simulink model "radarDFT"  (R2013a)
settings: Solver=ode45  StartTime=0.0  StopTime=90  RelTol=1e-3
PostLoadFcn:
  | bps_model_init(gcs);
undefined symbols (not defined in the file): xlipgetpartsetting
libraries: xbsIndex_r4 x69, xps_library x25, mbee4_library x4
(part 3 of 3)

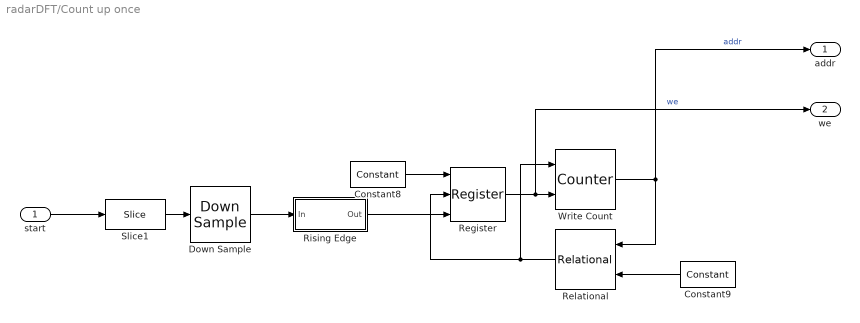
== system radarDFT/Count up once ==
  start : Inport
  Constant8 : xbsIndex_r4/Constant  const=1  gui_display_data_type=Fixed-point  arith_type=Boolean  n_bits=1  bin_pt=0  preci_type=Single  exp_width=8  frac_width=24  explicit_period=off  period=1  equ=P=C  opselect=C  inp2=PCIN>>17  opr=+  inp1=P  carry=CIN  dbl_ovrd=off  block_type=constant
  Constant9 : xbsIndex_r4/Constant  const=str2num(get_param('radarDFT/numofsamples','value'))-2  gui_display_data_type=Fixed-point  arith_type=Unsigned  n_bits=19  bin_pt=0  preci_type=Single  exp_width=8  frac_width=24  explicit_period=off  period=1e-8  equ=P=C  opselect=C  inp2=PCIN>>17  opr=+  inp1=P  carry=CIN  dbl_ovrd=off  block_type=constant
  Down Sample : xbsIndex_r4/Down Sample  sample_ratio=fix(250000/str2num(get_param('radarDFT/sampfreq(kHz)','value')))  sample_phase="Last Value of Frame  (most efficient)"  en=off  latency=1  dbl_ovrd=off  block_type=dsamp
  Register : xbsIndex_r4/Register  init=0  rst=on  en=on  dbl_ovrd=off  block_type=register
  Relational : xbsIndex_r4/Relational  mode=a=b  en=off  latency=1  dbl_ovrd=off  block_type=relational
      settings: block_version=10.1.3
  Rising Edge : Subsystem
  Slice1 : xbsIndex_r4/Slice  nbits=1  boolean_output=on  mode=Lower Bit Location + Width  bit1=0  base1=MSB of Input  bit0=0  base0=LSB of Input  dbl_ovrd=off  block_type=slice
      settings: infoedit="Extracts a given range of bits from each input sample and presents it at the output.  The output type is ordinarily unsigned with binary point at zero, but can be Boolean when the slice is one bit wide.<P><P>Hardware notes: In hardware this block costs nothing."  block_version=10.1.3
  Write Count : xbsIndex_r4/Counter  cnt_type=Free Running  cnt_to=Inf  operation=Up  start_count=0  cnt_by_val=1  arith_type=Unsigned  n_bits=19  bin_pt=0  load_pin=off  rst=on  en=on  explicit_period=on  period=fix(250000/str2num(get_param('radarDFT/sampfreq(kHz)','value')))  dbl_ovrd=off  use_behavioral_HDL=off  implementation=Fabric  use_rpm=off  block_type=counter
  addr : Outport
  we : Outport  Port=2
  wires:
  Write Count/1 -> addr/1, Relational/1  "addr"
  Relational/1 -> Write Count/1, Register/2
  Constant9/1 -> Relational/2
  Register/1 -> we/1, Write Count/2  "we"
  Rising Edge/1(Out) -> Register/3
  Slice1/1 -> Down Sample/1
  Constant8/1 -> Register/1
  start/1 -> Slice1/1
  Down Sample/1 -> Rising Edge/1(In)

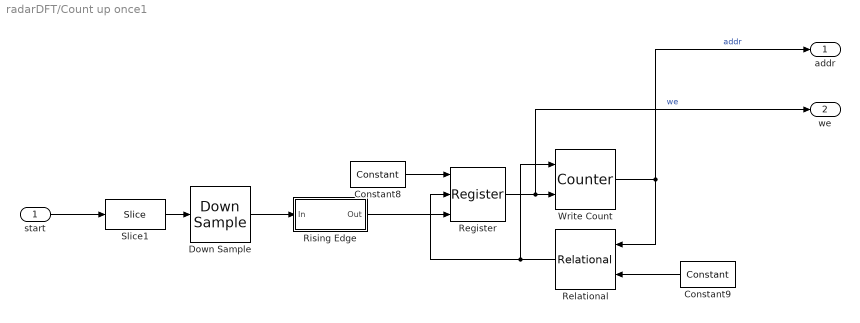
== system radarDFT/Count up once1 ==
  start : Inport
  Constant8 : xbsIndex_r4/Constant  const=1  gui_display_data_type=Boolean  arith_type=Boolean  n_bits=1  bin_pt=0  preci_type=Single  exp_width=8  frac_width=24  explicit_period=off  period=1  equ=P=C  opselect=C  inp2=PCIN>>17  opr=+  inp1=P  carry=CIN  dbl_ovrd=off  block_type=constant
  Constant9 : xbsIndex_r4/Constant  const=2^16-2  gui_display_data_type=Fixed-point  arith_type=Unsigned  n_bits=16  bin_pt=0  preci_type=Single  exp_width=8  frac_width=24  explicit_period=off  period=1e-8  equ=P=C  opselect=C  inp2=PCIN>>17  opr=+  inp1=P  carry=CIN  dbl_ovrd=off  block_type=constant
  Down Sample : xbsIndex_r4/Down Sample  sample_ratio=fix(250000/30)  sample_phase="Last Value of Frame  (most efficient)"  en=off  latency=1  dbl_ovrd=off  block_type=dsamp
  Register : xbsIndex_r4/Register  init=0  rst=on  en=on  dbl_ovrd=off  block_type=register
  Relational : xbsIndex_r4/Relational  mode=a=b  en=off  latency=1  dbl_ovrd=off  block_type=relational
      settings: block_version=10.1.3
  Rising Edge : Subsystem
  Slice1 : xbsIndex_r4/Slice  nbits=1  boolean_output=on  mode=Lower Bit Location + Width  bit1=0  base1=MSB of Input  bit0=0  base0=LSB of Input  dbl_ovrd=off  block_type=slice
      settings: infoedit="Extracts a given range of bits from each input sample and presents it at the output.  The output type is ordinarily unsigned with binary point at zero, but can be Boolean when the slice is one bit wide.<P><P>Hardware notes: In hardware this block costs nothing."  block_version=10.1.3
  Write Count : xbsIndex_r4/Counter  cnt_type=Free Running  cnt_to=Inf  operation=Up  start_count=0  cnt_by_val=1  arith_type=Unsigned  n_bits=16  bin_pt=0  load_pin=off  rst=on  en=on  explicit_period=on  period=fix(250000/30)  dbl_ovrd=off  use_behavioral_HDL=off  implementation=Fabric  use_rpm=off  block_type=counter
  addr : Outport
  we : Outport  Port=2
  wires:
  Write Count/1 -> addr/1, Relational/1  "addr"
  Relational/1 -> Write Count/1, Register/2
  Constant9/1 -> Relational/2
  Register/1 -> we/1, Write Count/2  "we"
  Rising Edge/1(Out) -> Register/3
  Slice1/1 -> Down Sample/1
  Constant8/1 -> Register/1
  start/1 -> Slice1/1
  Down Sample/1 -> Rising Edge/1(In)

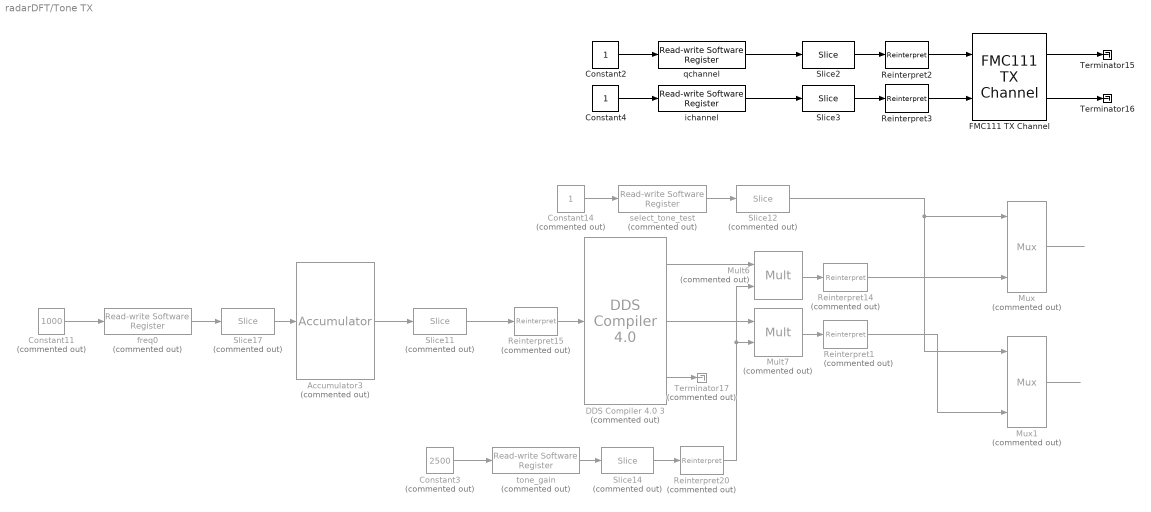
== system radarDFT/Tone TX ==
  Accumulator3 : xbsIndex_r4/Accumulator  Commented=on  operation=Add  n_bits=24  overflow=Wrap  scale=1  rst=off  infoeditControl=reset for floating point data type must be asserted for a minimum of 2 cycles  hasbypass=on  en=off  latency=0  dbl_ovrd=off  msb_inp=100  msb=100  lsb=-100  use_behavioral_HDL=on  implementation=Fabric  block_type=accum
  Constant11 : Constant  Commented=on  Value=1000
  Constant14 : Constant  Commented=on
  Constant2 : Constant
  Constant3 : Constant  Commented=on  Value=2500
  Constant4 : Constant
  DDS Compiler 4.0 3 : xbsIndex_r4/DDS Compiler 4.0   Commented=on  partspresent=SIN_COS_LUT_only  dds_clock_rate=100  channels=1  parameter_entry=Hardware_Parameters  spurious_free_dynamic_range=36  frequency_resolution=0.4  noise_shaping=None  phase_width=16  output_width=16  output_selection=Sine_and_Cosine  negative_sine=off  negative_cosine=off  amplitude_mode=Full_Range  memory_type=Distributed_ROM  optimization_goal=Auto  dsp48_use=Minimal  latency_configuration=Auto  latency=6  has_phase_out=on  sclr_pin=off  clock_enable=off  rfd=off  rdy=off  channel_pin=off  explicit_period=off  period=1  phase_increment=Fixed  output_frequency1=0  output_frequency2=0  output_frequency3=0  output_frequency4=0  output_frequency5=0  output_frequency6=0  output_frequency7=0  output_frequency8=0  output_frequency9=0  output_frequency10=0  output_frequency11=0  output_frequency12=0  output_frequency13=0  output_frequency14=0  output_frequency15=0  output_frequency16=0  pinc1='0'  pinc2='0'  pinc3='0'  pinc4='0'  pinc5='0'  pinc6='0'  pinc7='0'  pinc8='0'  pinc9='0'  pinc10='0'  pinc11='0'  pinc12='0'  pinc13='0'  pinc14='0'  pinc15='0'  pinc16='0'  phase_offset=None  phase_offset_angles1=0  phase_offset_angles2=0  phase_offset_angles3=0  phase_offset_angles4=0  phase_offset_angles5=0  phase_offset_angles6=0  phase_offset_angles7=0  phase_offset_angles8=0  phase_offset_angles9=0  phase_offset_angles10=0  phase_offset_angles11=0  phase_offset_angles12=0  phase_offset_angles13=0  phase_offset_angles14=0  phase_offset_angles15=0  phase_offset_angles16=0  poff1='0'  poff2='0'  poff3='0'  poff4='0'  poff5='0'  poff6='0'  poff7='0'  poff8='0'  poff9='0'  poff10='0'  poff11='0'  poff12='0'  poff13='0'  poff14='0'  poff15='0'  poff16='0'  por_mode=false  gui_behaviour=Sysgen  ip_name=DDS Compiler  ip_version=4.0  dsptool_ready=true  wrapper_available=true  port_translation_map={ 'ce' => 'en', 'sclr' => 'rst' }  ipcore_xco_need_fpga_part=true  ipcore_fpga_part=xlipgetpartsetting(gcb, {'virtex4', 'xc4vsx35', '-10', 'ff668'})  ipcore_usecache=true  ipcore_useipmodelcache=true  ipcore_verbose=false  block_type=dds_compiler_v4_0
  FMC111 TX Channel : mbee4_library/FMC111 TX Channel  Tag=xps:fmc111_tx  channel_number=1  arith_type=Signed  bitwidth=16  bin_pt=0  sample_period=1  update=off
  Mult6 : xbsIndex_r4/Mult  Commented=on  precision=User Defined  arith_type="Signed  (2's comp)"  n_bits=16  bin_pt=15  quantization="Round  (unbiased: +/- Inf)"  overflow=Saturate  en=off  latency=3  dbl_ovrd=off  use_behavioral_HDL=off  opt=Speed  use_embedded=on  optimum_pipeline=off  pipeline=on  use_rpm=on  placement_style=Triangular  block_type=mult
  Mult7 : xbsIndex_r4/Mult  Commented=on  precision=User Defined  arith_type="Signed  (2's comp)"  n_bits=16  bin_pt=15  quantization="Round  (unbiased: +/- Inf)"  overflow=Saturate  en=off  latency=3  dbl_ovrd=off  use_behavioral_HDL=off  opt=Speed  use_embedded=on  optimum_pipeline=off  pipeline=on  use_rpm=on  placement_style=Triangular  block_type=mult
  Mux : xbsIndex_r4/Mux  Commented=on  inputs=2  en=off  latency=0  precision=Full  arith_type=Unsigned  n_bits=16  bin_pt=14  quantization=Truncate  overflow=Wrap  dbl_ovrd=off  block_type=mux
  Mux1 : xbsIndex_r4/Mux  Commented=on  inputs=2  en=off  latency=0  precision=Full  arith_type=Unsigned  n_bits=16  bin_pt=14  quantization=Truncate  overflow=Wrap  dbl_ovrd=off  block_type=mux
  Reinterpret1 : xbsIndex_r4/Reinterpret  Commented=on  force_arith_type=on  arith_type="Signed  (2's comp)"  force_bin_pt=on  bin_pt=0  block_type=reinterpret
  Reinterpret14 : xbsIndex_r4/Reinterpret  Commented=on  force_arith_type=on  arith_type="Signed  (2's comp)"  force_bin_pt=on  bin_pt=0  block_type=reinterpret
  Reinterpret15 : xbsIndex_r4/Reinterpret  Commented=on  force_arith_type=off  arith_type=Unsigned  force_bin_pt=on  bin_pt=16  block_type=reinterpret
  Reinterpret2 : xbsIndex_r4/Reinterpret  force_arith_type=on  arith_type="Signed  (2's comp)"  force_bin_pt=on  bin_pt=0  block_type=reinterpret
  Reinterpret20 : xbsIndex_r4/Reinterpret  Commented=on  force_arith_type=on  arith_type=Unsigned  force_bin_pt=on  bin_pt=11  block_type=reinterpret
  Reinterpret3 : xbsIndex_r4/Reinterpret  force_arith_type=on  arith_type="Signed  (2's comp)"  force_bin_pt=on  bin_pt=0  block_type=reinterpret
  Slice11 : xbsIndex_r4/Slice  Commented=on  nbits=16  boolean_output=off  mode=Upper Bit Location + Width  bit1=0  base1=MSB of Input  bit0=0  base0=LSB of Input  dbl_ovrd=off  block_type=slice
  Slice12 : xbsIndex_r4/Slice  Commented=on  nbits=1  boolean_output=on  mode=Lower Bit Location + Width  bit1=0  base1=MSB of Input  bit0=0  base0=LSB of Input  dbl_ovrd=off  block_type=slice
  Slice14 : xbsIndex_r4/Slice  Commented=on  nbits=12  boolean_output=off  mode=Lower Bit Location + Width  bit1=0  base1=MSB of Input  bit0=0  base0=LSB of Input  dbl_ovrd=off  block_type=slice
  Slice17 : xbsIndex_r4/Slice  Commented=on  nbits=24  boolean_output=off  mode=Lower Bit Location + Width  bit1=0  base1=MSB of Input  bit0=0  base0=LSB of Input  dbl_ovrd=off  block_type=slice
  Slice2 : xbsIndex_r4/Slice  nbits=16  boolean_output=off  mode=Lower Bit Location + Width  bit1=0  base1=MSB of Input  bit0=0  base0=LSB of Input  dbl_ovrd=off  block_type=slice
  Slice3 : xbsIndex_r4/Slice  nbits=16  boolean_output=off  mode=Lower Bit Location + Width  bit1=0  base1=MSB of Input  bit0=0  base0=LSB of Input  dbl_ovrd=off  block_type=slice
  Terminator15 : Terminator
  Terminator16 : Terminator
  Terminator17 : Terminator  Commented=on
  freq0 : xps_library/Read-write Software Register  Tag=xps:sw_reg  Commented=on  io_dir=From Processor  use_strobe=off  arith_type=Unsigned  bitwidth=32  bin_pt=0  sample_period=1  update=off
  ichannel : xps_library/Read-write Software Register  Tag=xps:sw_reg  io_dir=From Processor  use_strobe=off  arith_type=Unsigned  bitwidth=32  bin_pt=0  sample_period=1  update=off
  qchannel : xps_library/Read-write Software Register  Tag=xps:sw_reg  io_dir=From Processor  use_strobe=off  arith_type=Unsigned  bitwidth=32  bin_pt=0  sample_period=1  update=off
  select_tone_test : xps_library/Read-write Software Register  Tag=xps:sw_reg  Commented=on  io_dir=From Processor  use_strobe=off  arith_type=Unsigned  bitwidth=32  bin_pt=0  sample_period=1  update=off
  tone_gain : xps_library/Read-write Software Register  Tag=xps:sw_reg  Commented=on  io_dir=From Processor  use_strobe=off  arith_type=Unsigned  bitwidth=32  bin_pt=0  sample_period=1  update=off
  wires:
  Accumulator3/1 -> Slice11/1
  select_tone_test/1 -> Slice12/1
  Mult7/1 -> Reinterpret1/1
  tone_gain/1 -> Slice14/1
  Reinterpret20/1 -> Mult6/2, Mult7/2
  Constant3/1 -> tone_gain/1
  qchannel/1 -> Slice2/1
  FMC111 TX Channel/1 -> Terminator15/1
  DDS Compiler 4.0 3/2 -> Mult7/1
  DDS Compiler 4.0 3/3 -> Terminator17/1
  Reinterpret1/1 -> Mux1/3
  Slice2/1 -> Reinterpret2/1
  Reinterpret3/1 -> FMC111 TX Channel/2
  freq0/1 -> Slice17/1
  Constant11/1 -> freq0/1
  Mult6/1 -> Reinterpret14/1
  Slice17/1 -> Accumulator3/1
  Slice12/1 -> Mux/1, Mux1/1
  Mux/1 -> ?
  Constant4/1 -> ichannel/1
  Slice3/1 -> Reinterpret3/1
  Mux1/1 -> ?
  Reinterpret2/1 -> FMC111 TX Channel/1
  Constant2/1 -> qchannel/1
  Constant14/1 -> select_tone_test/1
  Reinterpret15/1 -> DDS Compiler 4.0 3/1
  Reinterpret14/1 -> Mux/3
  Slice11/1 -> Reinterpret15/1
  DDS Compiler 4.0 3/1 -> Mult6/1
  ichannel/1 -> Slice3/1
  Slice14/1 -> Reinterpret20/1
  FMC111 TX Channel/2 -> Terminator16/1

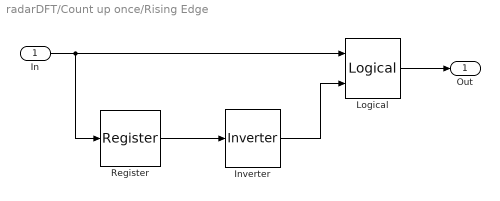
== system radarDFT/Count up once/Rising Edge ==
  In : Inport
  Inverter : xbsIndex_r4/Inverter  en=off  latency=0  dbl_ovrd=off  block_type=inv
  Logical : xbsIndex_r4/Logical  logical_function=AND  inputs=2  en=off  latency=0  precision=Full  arith_type=Unsigned  n_bits=16  bin_pt=0  align_bp=on  dbl_ovrd=off  block_type=logical
  Register : xbsIndex_r4/Register  init=0  rst=off  en=off  dbl_ovrd=off  block_type=register
  Out : Outport
  wires:
  Logical/1 -> Out/1
  Inverter/1 -> Logical/2
  Register/1 -> Inverter/1
  In/1 -> Logical/1, Register/1

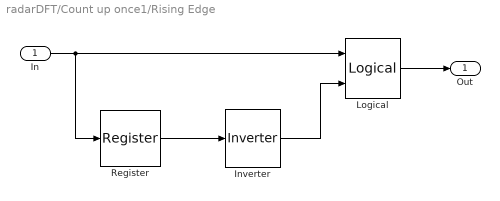
== system radarDFT/Count up once1/Rising Edge ==
  In : Inport
  Inverter : xbsIndex_r4/Inverter  en=off  latency=0  dbl_ovrd=off  block_type=inv
  Logical : xbsIndex_r4/Logical  logical_function=AND  inputs=2  en=off  latency=0  precision=Full  arith_type=Unsigned  n_bits=16  bin_pt=0  align_bp=on  dbl_ovrd=off  block_type=logical
  Register : xbsIndex_r4/Register  init=0  rst=off  en=off  dbl_ovrd=off  block_type=register
  Out : Outport
  wires:
  Logical/1 -> Out/1
  Inverter/1 -> Logical/2
  Register/1 -> Inverter/1
  In/1 -> Logical/1, Register/1
